simulink model "simulation_ACC_test"  (R2018b)
settings: Solver=ode2  StartTime=0.0  StopTime=90  FixedStep=0.4  RelTol=1e-3
undefined symbols (not defined in the file or in its folder): Delta_T, DiscIntNeverNeededParam, lead_bot_vel_vari, lead_bot_vel_vari_const, sigbuilder_block, timebpt
libraries: commchan3 x11, visionstatistics x4, simulink x3
(part 1 of 3)
settings Model: Creator=UWEcocar  LastModifiedBy=UWEcocar

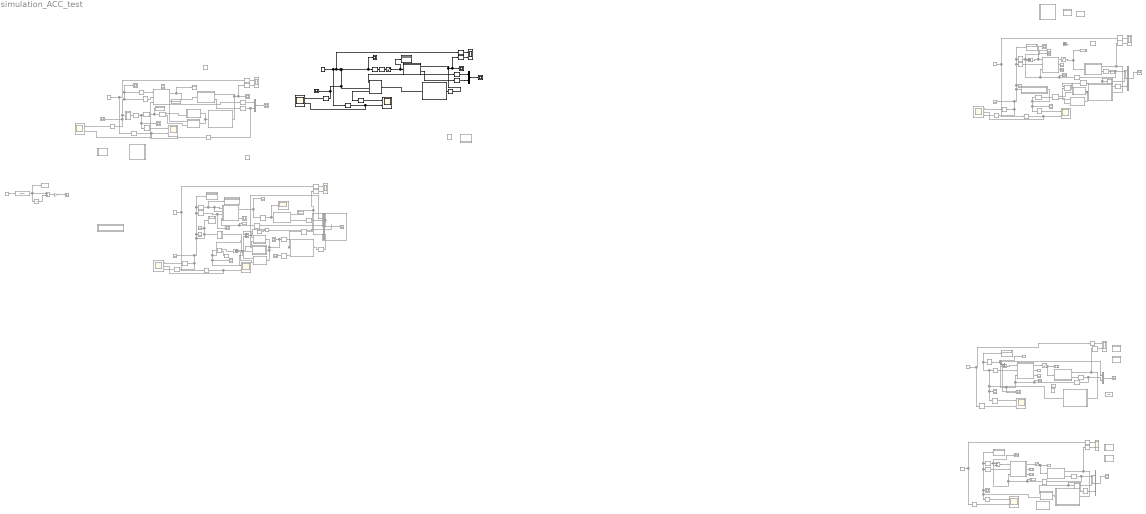
== system simulation_ACC_test ==
  1-D Kalman Filter : Subsystem  Commented=on
  1-D Kalman Filter1 : Subsystem  Commented=on
  1-D Kalman Filter2 : Subsystem  Commented=on
  1-D Kalman Filter3 : Subsystem  Commented=on
  2-D Mean1 : visionstatistics/2-D Mean  Commented=on  run=off  reset_popup=None  directionMode=Each row  dimension=1  treatSBRowAsCol=on  roiEnable=off  roiType=Rectangles  roiPortion=Entire ROI  roiOutput=Individual statistics for each ROI  roiFlag=off  outputDataTypeStr=Inherit: Same as accumulator  outputLastDataTypeStr=Inherit: Same as accumulator  outputMin=[]  outputMax=[]  accumMode=Binary point scaling  accumWordLength=32  accumFracLength=0  accumDataTypeStr=fixdt([],32,0)  accumLastDataTypeStr=fixdt([],32,0)  roundingMode=Floor  overflowMode=off
      settings: SourceProductName=Computer Vision System Toolbox  SourceProductBaseCode=VP
  2-D Mean2 : visionstatistics/2-D Mean  Commented=on  run=off  reset_popup=None  directionMode=Each row  dimension=1  treatSBRowAsCol=on  roiEnable=off  roiType=Rectangles  roiPortion=Entire ROI  roiOutput=Individual statistics for each ROI  roiFlag=off  outputDataTypeStr=Inherit: Same as accumulator  outputLastDataTypeStr=Inherit: Same as accumulator  outputMin=[]  outputMax=[]  accumMode=Binary point scaling  accumWordLength=32  accumFracLength=0  accumDataTypeStr=fixdt([],32,0)  accumLastDataTypeStr=fixdt([],32,0)  roundingMode=Floor  overflowMode=off
      settings: SourceProductName=Computer Vision System Toolbox  SourceProductBaseCode=VP
  2-D Mean3 : visionstatistics/2-D Mean  Commented=on  run=off  reset_popup=None  directionMode=Each row  dimension=1  treatSBRowAsCol=on  roiEnable=off  roiType=Rectangles  roiPortion=Entire ROI  roiOutput=Individual statistics for each ROI  roiFlag=off  outputDataTypeStr=Inherit: Same as accumulator  outputLastDataTypeStr=Inherit: Same as accumulator  outputMin=[]  outputMax=[]  accumMode=Binary point scaling  accumWordLength=32  accumFracLength=0  accumDataTypeStr=fixdt([],32,0)  accumLastDataTypeStr=fixdt([],32,0)  roundingMode=Floor  overflowMode=off
      settings: SourceProductName=Computer Vision System Toolbox  SourceProductBaseCode=VP
  Add : Sum  Commented=on
  Add1 : Sum  Commented=on
  Add2 : Sum  Commented=on  Inputs=+-
  Bus Creator : BusCreator  Inputs=2
  Bus Creator1 : BusCreator  Commented=on  Inputs=2
  Bus Creator2 : BusCreator  Commented=on  Inputs=3
  Bus Creator3 : BusCreator  Commented=on  Inputs=3
  Bus Creator4 : BusCreator  Commented=on  Inputs=3
  Bus Creator5 : BusCreator  Commented=on  Inputs=2
  Camera Sensor1 : Subsystem  Commented=on
  Camera Sensor2 : Subsystem  Commented=on
  Camera Sensor3 : Subsystem  Commented=on
  Camera Sensor4 : Subsystem  Commented=on
  Constant : Constant  Value=[0.4;0]  VectorParams1D=off
  Constant{1..4,7} (5 alike) : Constant  Commented=on  Value=[0.4;0]  VectorParams1D=off
  Constant5 : Constant  Commented=on  Value=0.5
  Constant6 : Constant  Commented=on  Value=0.5
  Delay : Delay  DelayLength=1
  Delay1 : Delay  Commented=on
  Delay2 : Delay  Commented=on
  Delay3 : Delay  Commented=on  DelayLength=1
  Discrete Transfer Fcn : DiscreteTransferFcn  Commented=on  Denominator=[1 0.4]
  Discrete Transfer Fcn1 : DiscreteTransferFcn  Commented=on  Denominator=[1 0.4]
  Discrete Derivative : simulink/Discrete/Discrete Derivative  Commented=on  gainval=1.0  ICPrevScaledInput=0.0  OutMin=[]  OutMax=[]  OutDataType=fixdt(1, 16)  OutScaling=2^-10  DoSatur=off
  Discrete PID Controller : simulink/Continuous/PID Controller  Controller=PI  Form=Parallel  TimeDomain=Discrete-time  SampleTime=-1  IntegratorMethod=Forward Euler  FilterMethod=Forward Euler  ControllerParametersSource=internal  P=0.5  I=0.01  D=0  UseFilter=on  N=100  TunerSelectOption=Transfer Function Based (PID Tuner App)  InitialConditionSource=internal  InitialConditionForIntegrator=0  InitialConditionForFilter=0  DifferentiatorICPrevScaledInput=0  ExternalReset=none  TrackingMode=off  Kt=1  LimitOutput=on  UpperSaturationLimit=0.2  LowerSaturationLimit=-0.2  LinearizeAsGain=off  AntiWindupMode=clamping  Kb=1  POutMin=[]  POutMax=[]  IOutMin=[]  IOutMax=[]  DOutMin=[]  DOutMax=[]  NOutMin=[]  NOutMax=[]  SumOutMin=[]  SumOutMax=[]  SaturationOutMin=[]  SaturationOutMax=[]  PParamMin=[]  PParamMax=[]  IParamMin=[]  IParamMax=[]  DParamMin=[]  DParamMax=[]  NParamMin=[]  NParamMax=[]  KbParamMin=[]  KbParamMax=[]  KtParamMin=[]  KtParamMax=[]  KbOutMin=[]  KbOutMax=[]  KtOutMin=[]  KtOutMax=[]  IntegratorOutMin=[]  IntegratorOutMax=[]  FilterOutMin=[]  FilterOutMax=[]  SumI1OutMin=[]  SumI1OutMax=[]  SumI2OutMin=[]  SumI2OutMax=[]  SumI3OutMin=[]  SumI3OutMax=[]  SumI4OutMin=[]  SumI4OutMax=[]  SumDOutMin=[]  SumDOutMax=[]  DifferentiatorOutMin=[]  DifferentiatorOutMax=[]  FilterDiffOutCoefMin=[]  FilterDiffOutCoefMax=[]  ReciprocalOutMin=[]  ReciprocalOutMax=[]  SumDenOutMin=[]  SumDenOutMax=[]  SumNumOutMin=[]  SumNumOutMax=[]  DivideOutMin=[]  DivideOutMax=[]  IntegratorContinuousStateAttributes=''  IntegratorStateMustResolveToSignalObject=off  IntegratorRTWStateStorageClass=Auto  FilterContinuousStateAttributes=''  FilterStateMustResolveToSignalObject=off  FilterRTWStateStorageClass=Auto  ParallelPVariant=InternalParameters  IdealPVariant=Disabled  IVariant=InternalParameters  DVariant=Disabled  IntegratorVariant=Discrete  SatVariant=Enabled  AWVariant=DiscClampingParallel  PCopyVariant=Disabled  TRVariant=Disabled  FdbkBlocksVariant=Forward  IdealPFdbkVariant=Disabled  SatFdbkVariant=Disabled  DerivativeFilterVariant=Disabled  NVariant=Disabled  NCopyVariant=Disabled_SignalSpec  FilterICVariant=Disabled  IntegratorICVariant=InternalICs  ExternalResetVariant=Disabled  TRSumVariant=Passthrough  SumFdbkVariant=Disabled  SumVariant=Sum_PI
  Discrete PID motor Controller2 : simulink/Continuous/PID Controller  Commented=on  Controller=PI  Form=Parallel  TimeDomain=Discrete-time  SampleTime=-1  IntegratorMethod=Forward Euler  FilterMethod=Forward Euler  ControllerParametersSource=internal  P=0.7813  I=0.0153  D=0  UseFilter=on  N=100  TunerSelectOption=Transfer Function Based (PID Tuner App)  InitialConditionSource=internal  InitialConditionForIntegrator=0  InitialConditionForFilter=0  DifferentiatorICPrevScaledInput=0  ExternalReset=none  TrackingMode=off  Kt=1  LimitOutput=on  UpperSaturationLimit=0.2  LowerSaturationLimit=-0.2  LinearizeAsGain=off  AntiWindupMode=clamping  Kb=1  POutMin=[]  POutMax=[]  IOutMin=[]  IOutMax=[]  DOutMin=[]  DOutMax=[]  NOutMin=[]  NOutMax=[]  SumOutMin=[]  SumOutMax=[]  SaturationOutMin=[]  SaturationOutMax=[]  PParamMin=[]  PParamMax=[]  IParamMin=[]  IParamMax=[]  DParamMin=[]  DParamMax=[]  NParamMin=[]  NParamMax=[]  KbParamMin=[]  KbParamMax=[]  KtParamMin=[]  KtParamMax=[]  KbOutMin=[]  KbOutMax=[]  KtOutMin=[]  KtOutMax=[]  IntegratorOutMin=[]  IntegratorOutMax=[]  FilterOutMin=[]  FilterOutMax=[]  SumI1OutMin=[]  SumI1OutMax=[]  SumI2OutMin=[]  SumI2OutMax=[]  SumI3OutMin=[]  SumI3OutMax=[]  SumI4OutMin=[]  SumI4OutMax=[]  SumDOutMin=[]  SumDOutMax=[]  DifferentiatorOutMin=[]  DifferentiatorOutMax=[]  FilterDiffOutCoefMin=[]  FilterDiffOutCoefMax=[]  ReciprocalOutMin=[]  ReciprocalOutMax=[]  SumDenOutMin=[]  SumDenOutMax=[]  SumNumOutMin=[]  SumNumOutMax=[]  DivideOutMin=[]  DivideOutMax=[]  IntegratorContinuousStateAttributes=''  IntegratorStateMustResolveToSignalObject=off  IntegratorRTWStateStorageClass=Auto  FilterContinuousStateAttributes=''  FilterStateMustResolveToSignalObject=off  FilterRTWStateStorageClass=Auto  ParallelPVariant=InternalParameters  IdealPVariant=Disabled  IVariant=InternalParameters  DVariant=Disabled  IntegratorVariant=Discrete  SatVariant=Enabled  AWVariant=DiscClampingParallel  PCopyVariant=Disabled  TRVariant=Disabled  FdbkBlocksVariant=Forward  IdealPFdbkVariant=Disabled  SatFdbkVariant=Disabled  DerivativeFilterVariant=Disabled  NVariant=Disabled  NCopyVariant=Disabled_SignalSpec  FilterICVariant=Disabled  IntegratorICVariant=InternalICs  ExternalResetVariant=Disabled  TRSumVariant=Passthrough  SumFdbkVariant=Disabled  SumVariant=Sum_PI
  Display{,1..12,14..26} (26 alike) : Display  Commented=on
  Display13 : Display
  Ego vehicle Kinamatics : Subsystem
  Ego vehicle Kinamatics1 : Subsystem  Commented=on
  Ego vehicle Kinamatics2 : Subsystem  Commented=on
  Ego vehicle Kinamatics3 : Subsystem  Commented=on
  Ego vehicle Kinamatics4 : Subsystem  Commented=on
  Ego vehicle Kinamatics5 : Subsystem  Commented=on
  Gain : Gain  Commented=on  Gain=1/Delta_T
  LDS sensor1 : Subsystem  Commented=on
  LDS sensor2 : Subsystem  Commented=on
  LDS sensor3 : Subsystem  Commented=on
  LDS sensor4 : Subsystem  Commented=on
  Lead vehicle trajectory : Subsystem
  Lead vehicle trajectory1 : Subsystem  Commented=on
  Lead vehicle trajectory2 : Subsystem  Commented=on
  Lead vehicle trajectory3 : Subsystem  Commented=on
  Lead vehicle trajectory4 : Subsystem  Commented=on
  Lead vehicle trajectory5 : Subsystem  Commented=on
  MATLAB Function1 : MATLAB Function  Commented=on  TreatAsAtomicUnit=on
  MATLAB Function10 : MATLAB Function  Commented=on  TreatAsAtomicUnit=on
  MATLAB Function11 : MATLAB Function  Commented=on  TreatAsAtomicUnit=on
  MATLAB Function12 : MATLAB Function  Commented=on  TreatAsAtomicUnit=on
  MATLAB Function13 : MATLAB Function  Commented=on  TreatAsAtomicUnit=on
  MATLAB Function2 : MATLAB Function  Commented=on  TreatAsAtomicUnit=on
  MATLAB Function3 : MATLAB Function  Commented=on  TreatAsAtomicUnit=on
  MATLAB Function4 : MATLAB Function  Commented=on  TreatAsAtomicUnit=on
  MATLAB Function5 : MATLAB Function  Commented=on  TreatAsAtomicUnit=on
  MATLAB Function6 : MATLAB Function  Commented=on  TreatAsAtomicUnit=on
  MATLAB Function7 : MATLAB Function  Commented=on  TreatAsAtomicUnit=on
  MATLAB Function8 : MATLAB Function  Commented=on  TreatAsAtomicUnit=on
  MATLAB Function9 : MATLAB Function  Commented=on  TreatAsAtomicUnit=on
  Matrix Concatenate1 : Concatenate  Commented=on  Mode=Multidimensional array  ConcatenateDimension=2
  Matrix Concatenate2 : Concatenate  Commented=on  Mode=Multidimensional array  ConcatenateDimension=2
  Matrix Concatenate3 : Concatenate  Commented=on  Mode=Multidimensional array  ConcatenateDimension=2
  Memory : Memory  Commented=on
  Multiply : Product  Commented=on
  Multiply1 : Product  Commented=on
  New_1d_kalman_filter : Subsystem  Commented=on
  New_1d_kalman_filter2 : Subsystem  Commented=on
  Saturation : Saturate  Commented=on  UpperLimit=0.2  LowerLimit=-0.2
  Saturation1 : Saturate  Commented=on  UpperLimit=0.2  LowerLimit=-0.2
  Saturation2 : Saturate  UpperLimit=0.2  LowerLimit=0
  Saturation3 : Saturate  Commented=on  UpperLimit=0.2  LowerLimit=0
  Scope{,2..3,5} (4 alike) : Scope
  Scope1 : Scope  NumInputPorts=2
  Scope{7,10,12,16..17,19,25..26,32,40,43,46} (12 alike) : Scope  Commented=on  NumInputPorts=2
  Scope{6,9,11,13..15,18,20..22,24,27..29,31,33..39,41..42,44..45,47} (27 alike) : Scope  Commented=on
  Scope23 : Scope  Commented=on  NumInputPorts=3
  Scope30 : Scope  Commented=on  NumInputPorts=3
  Scope4 : Scope  NumInputPorts=2
  Scope8 : Scope  NumInputPorts=2
  Selector{1..4,6..7,12} (7 alike) : Selector  InputPortWidth=2  IndexOptions=Index vector (dialog)  Indices=[1]  OutputSizes=1
  Selector{8..11,13..14,16..19,21..22,25,27..28,30..34,36,38..40,42..47,49..51,53..54,56} (36 alike) : Selector  Commented=on  InputPortWidth=2  IndexOptions=Index vector (dialog)  Indices=[1]  OutputSizes=1
  Selector{15,20,23..24,26,29,35,37,41,48,52,55} (12 alike) : Selector  Commented=on  InputPortWidth=2  IndexOptions=Index vector (dialog)  Indices=[2]  OutputSizes=1
  Selector5 : Selector  InputPortWidth=2  IndexOptions=Index vector (dialog)  Indices=[2]  OutputSizes=1
  Sensor Fusion : Subsystem
  Subtract{,1..3} (4 alike) : Sum  Commented=on  Inputs=+-
  Sum : Sum  Inputs=|-+
  Transfer Fcn : TransferFcn  Commented=on  Denominator=[4 1]
  Transfer Fcn1 : TransferFcn  Commented=on  Denominator=[0.2 1]
  Transport Delay{,1..2,4..5} (5 alike) : TransportDelay  Commented=on  DelayTime=0.8
  Transport Delay3 : TransportDelay  Commented=on  DelayTime=0.4
  Transport Delay9 : TransportDelay  Commented=on  DelayTime=0.4
  Unit Delay : UnitDelay  Commented=on  SampleTime=-1
  Unit Delay1 : UnitDelay  Commented=on  SampleTime=-1
  V_lead2 : Constant  Commented=on
  combined sensor4 : Subsystem  Commented=on
  wires:
  Sum/1 -> Scope2/1, Selector1/1
  Constant/1 -> Selector6/1, Selector2/1, Sum/1
  Selector1/1 -> Discrete PID Controller/1
  Selector3/1 -> Scope1/2
  Selector2/1 -> Scope1/1
  Selector5/1 -> Bus Creator/1  "lead vehicle speed"
  Selector4/1 -> Bus Creator/2  "ego vehicle speed"
  Bus Creator/1 -> Scope5/1
  Selector6/1 -> Scope4/2, Scope8/2  "safe distance = 0.4m"
  Selector7/1 -> Scope8/1  "relative distance measured by sensor"
  Selector14/1 -> Scope17/1  "relative distance measured by sensor"
  MATLAB Function4/1(accel_new) -> Saturation/1  "ego vehicle speed"
  Constant2/1 -> Selector13/1, Selector9/1
  Selector10/1 -> Scope10/2
  Selector13/1 -> Scope17/2  "safe distance = 0.4m"
  Bus Creator1/1 -> Scope14/1
  Selector9/1 -> Scope10/1
  Lead vehicle trajectory2/1(Lead vehicle traject. and ego vehicle state out) -> Display/1, Selector15/1, Selector8/1, Selector14/1, Scope15/1
  Selector8/1 -> MATLAB Function4/2(rel_posx)  "relative distance"
  Selector15/1 -> Scope16/1, Subtract/1, Display3/1, Bus Creator1/1  "lead velocity"
  MATLAB Function4/2(stat) -> Display1/1
  Ego vehicle Kinamatics/1(Output for sensor feedback) -> Delay/1, Selector3/1, Scope/1
  Ego vehicle Kinamatics/2(ego vehicle speed) -> Selector4/1
  Selector12/1 -> Scope4/1  "relative distance estimated by kalman filter through sensor"
  MATLAB Function4/3(x) -> Display2/1
  Ego vehicle Kinamatics2/2(ego vehicle speed) -> Selector11/1
  Ego vehicle Kinamatics2/1(Output for sensor feedback) -> Selector10/1, Lead vehicle trajectory2/1(ego vehicle input)
  Subtract/1 -> MATLAB Function4/1(rel_velx)  "relative velocity"
  Selector11/1 -> Transport Delay/1, Bus Creator1/2  "ego vehicle speed"
  Saturation/1 -> Display4/1, Ego vehicle Kinamatics2/1(Controller input (x; vx))
  Saturation1/1 -> Display10/1, Ego vehicle Kinamatics1/1(Controller input (x; vx))
  Selector17/1 -> Transport Delay1/1, Bus Creator2/2  "ego vehicle speed"
  Ego vehicle Kinamatics1/1(Output for sensor feedback) -> Selector16/1, Lead vehicle trajectory1/1(ego vehicle input)
  Selector21/1 -> MATLAB Function6/2(rel_posx)  "relative distance"
  MATLAB Function6/3(x) -> Display8/1
  Subtract1/1 -> MATLAB Function6/1(rel_velx)  "relative velocity"
  Bus Creator2/1 -> Scope9/1
  Ego vehicle Kinamatics1/2(ego vehicle speed) -> Selector17/1
  Selector22/1 -> Scope7/1
  Selector16/1 -> Scope7/2
  MATLAB Function6/1(accel_new) -> Saturation1/1  "ego vehicle speed"
  Selector18/1 -> Scope12/2  "safe distance = 0.4m"
  Selector20/1 -> Display9/1, Subtract1/1  "lead velocity"
  Selector19/1 -> Scope12/1  "relative distance measured by sensor with noise"
  MATLAB Function6/2(stat) -> Display7/1
  Constant1/1 -> Selector18/1, Selector22/1
  Camera Sensor1/2(Sensor Output) -> Selector19/1, Scope11/1, Display6/1, Selector20/1, Selector21/1
  Lead vehicle trajectory1/1(Lead vehicle traject. and ego vehicle state out) -> Camera Sensor1/1(Traject. input)
  Camera Sensor1/1(Act lead vehicle speed) -> Selector26/1, Selector25/1
  Transport Delay/1 -> MATLAB Function4/3(vel_egox), Scope16/2, Subtract/2, Display5/1
  Transport Delay1/1 -> Display11/1, MATLAB Function6/3(vel_egox), Subtract1/2
  Delay/1 -> Lead vehicle trajectory/1(ego vehicle input)
  Selector25/1 -> Bus Creator2/1  "estimated distance by sensor"
  Selector26/1 -> Bus Creator2/3  "lead vehicle speed"
  Selector38/1 -> MATLAB Function12/2(rel_posx)  "relative distance"
  Subtract3/1 -> Scope13/1, Display12/1, MATLAB Function12/1(rel_velx)  "relative velocity"
  MATLAB Function12/2(stat) -> Display21/1
  MATLAB Function12/1(accel_new) -> Saturation3/1  "ego vehicle speed"
  Selector41/1 -> Bus Creator4/3  "lead vehicle speed"
  Ego vehicle Kinamatics3/2(ego vehicle speed) -> Selector34/1
  Selector33/1 -> Scope26/2
  Selector37/1 -> Display23/1, Subtract3/1  "lead velocity"
  MATLAB Function12/3(x) -> Display22/1
  Selector34/1 -> Discrete Transfer Fcn/1
  Selector39/1 -> Scope26/1
  Bus Creator4/1 -> Scope27/1
  Transport Delay4/1 -> Display19/1, MATLAB Function12/3(vel_egox), Subtract3/2
  Lead vehicle trajectory4/1(Lead vehicle traject. and ego vehicle state out) -> LDS sensor3/1(Traject. input), Camera Sensor3/1(Traject. input)
  Selector40/1 -> Bus Creator4/1  "estimated distance by sensor"
  Ego vehicle Kinamatics3/1(Output for sensor feedback) -> Selector33/1, Lead vehicle trajectory4/1(ego vehicle input)
  Camera Sensor3/1(Act lead vehicle speed) -> Matrix Concatenate3/1
  Selector43/1 -> Scope30/2, Scope32/2  "safe distance = 0.4m"
  2-D Mean2/1 -> 1-D Kalman Filter1/1(Sensor Input), Scope31/1, Selector44/1
  Selector44/1 -> Scope32/1  "relative distance measured by sensor"
  Selector42/1 -> Scope30/1  "relative distance estimated kalman filter"
  Matrix Concatenate2/1 -> 2-D Mean2/1
  Constant4/1 -> Selector43/1, Selector39/1
  LDS sensor3/2(Sensor Output) -> Matrix Concatenate2/2
  Camera Sensor3/2(Sensor Output) -> Matrix Concatenate2/1
  LDS sensor3/1(Act lead vehicle speed) -> Matrix Concatenate3/2
  Matrix Concatenate3/1 -> 2-D Mean3/1
  2-D Mean3/1 -> Selector41/1, Selector40/1
  1-D Kalman Filter1/1(measurement and estimated velocity) -> Selector23/1, Selector42/1, Scope29/1, Scope28/1, Selector38/1, Selector37/1, Display20/1
  Discrete PID Controller/1 -> Saturation2/1
  Saturation3/1 -> Ego vehicle Kinamatics3/1(Controller input (x; vx)), Display18/1  "opt_cmd"
  Selector23/1 -> Scope30/3  "relative velocity estimated kalman filter"
  Subtract2/1 -> ?
  Discrete Transfer Fcn/1 -> Transport Delay4/1, Bus Creator4/2  "ego vehicle speed"
  Selector24/1 -> Scope23/3  "relative velocity estimated kalman filter"
  MATLAB Function9/1(accel_new) -> Transport Delay9/1, Scope18/1  "opt_cmd"
  Ego vehicle Kinamatics4/1(Output for sensor feedback) -> Transport Delay5/1, Selector27/1
  Selector45/1 -> Scope23/2, Scope25/2  "safe distance = 0.4m"
  Lead vehicle trajectory3/1(Lead vehicle traject. and ego vehicle state out) -> Selector35/1, Selector47/1, Selector48/1
  Camera Sensor2/2(Sensor Output) -> Add1/1
  Selector31/1 -> Scope19/1
  Transport Delay3/1 -> MATLAB Function9/4(vel_egox), Display16/1
  Constant3/1 -> Selector45/1, Selector31/1
  Selector30/1 -> Scope38/1, MATLAB Function9/3(rel_posx)  "relative distance"
  Camera Sensor2/1(sensor rel. distance) -> Add/1
  Selector36/1 -> Scope23/1  "relative distance estimated kalman filter"
  Bus Creator3/1 -> Scope20/1
  LDS sensor2/2(Sensor Output) -> Add1/2
  LDS sensor2/1(sensor rel. distance) -> Add/2
  Add/1 -> Multiply/1
  Multiply/1 -> ?  "estimated distance by sensor"
  Selector29/1 -> MATLAB Function9/2(rel_velx), MATLAB Function9/1(lead_velocity), Display26/1  "lead velocity"
  Selector27/1 -> Scope19/2
  Add1/1 -> Multiply1/1
  Selector35/1 -> Bus Creator3/3  "lead vehicle speed"
  Multiply1/1 -> Scope24/1  "relative distance measured by sensor"
  Selector28/1 -> Transport Delay3/1, Bus Creator3/2  "ego vehicle speed"
  Selector47/1 -> combined sensor4/1(Traject. input), LDS sensor2/1(Traject. input), Camera Sensor2/1(Traject. input), Scope33/1  "relative distance"
  Selector48/1 -> Scope34/1
  Constant5/1 -> Multiply/2
  Constant6/1 -> Multiply1/2
  MATLAB Function9/2(stat) -> Scope37/1
  Ego vehicle Kinamatics4/2(ego vehicle speed) -> Selector28/1  "ego vehicle speed"
  Transport Delay9/1 -> Scope36/1, Ego vehicle Kinamatics4/1(Controller input (x; vx))
  combined sensor4/1(sensor rel. distance) -> Bus Creator3/1  "estimated distance by sensor"
  combined sensor4/2(Sensor Output) -> New_1d_kalman_filter2/1(In1), Scope25/1  "relative distance measured by sensor"
  New_1d_kalman_filter2/1(Out1) -> Selector24/1, Selector36/1, Scope22/1, Scope21/1, Selector30/1, Selector29/1, Display17/1, Display14/1, Scope35/1  "matlab kalman"
  Transport Delay5/1 -> Lead vehicle trajectory3/1(ego vehicle input)
  LDS sensor4/2(Sensor Output) -> Matrix Concatenate1/1
  Selector46/1 -> Scope43/1  "relative distance estimated be kalman filter through sensor"
  Selector51/1 -> Delay3/1, Bus Creator5/2  "ego vehicle speed"
  Selector49/1 -> Scope40/1
  Selector53/1 -> Scope43/2, Scope46/2  "safe distance = 0.4m"
  Ego vehicle Kinamatics5/1(Output for sensor feedback) -> Lead vehicle trajectory5/1(ego vehicle input), Selector50/1, Scope39/1
  Selector52/1 -> Bus Creator5/1  "lead vehicle speed"
  Camera Sensor4/2(Sensor Output) -> Matrix Concatenate1/2
  Selector32/1 -> MATLAB Function13/2(rel_posx)
  Ego vehicle Kinamatics5/2(ego vehicle speed) -> Selector51/1
  Selector54/1 -> Scope46/1  "relative distance measured by sensor"
  Matrix Concatenate1/1 -> Display25/1, 2-D Mean1/1
  Bus Creator5/1 -> Scope44/1
  Selector50/1 -> Scope40/2
  Constant7/1 -> Selector53/1, Selector49/1
  Camera Sensor4/1(Act lead vehicle speed) -> Selector52/1
  Lead vehicle trajectory5/1(Lead vehicle traject. and ego vehicle state out) -> LDS sensor4/1(Traject. input), Camera Sensor4/1(Traject. input)
  Selector55/1 -> MATLAB Function13/1(rel_velx)  "relative velocity estimated by kalman"
  MATLAB Function13/2(stat) -> Display24/1
  New_1d_kalman_filter/1(Out1) -> Selector32/1, Selector55/1, Scope41/1, Selector46/1, Scope42/1
  2-D Mean1/1 -> Selector56/1, Selector54/1, Scope45/1
  Selector56/1 -> New_1d_kalman_filter/1(In1)
  Saturation2/1 -> Display13/1, Ego vehicle Kinamatics/1(Controller input (x; vx))
  Sensor Fusion/3(kalman out) -> Sum/2, Scope3/1, Selector12/1
  Lead vehicle trajectory/1(Lead vehicle traject. and ego vehicle state out) -> Sensor Fusion/1(simulated input)
  Sensor Fusion/1(lead vehicle speed) -> Selector5/1
  Sensor Fusion/4(sensor out) -> Selector7/1
  MATLAB Function13/1(accel_new) -> Ego vehicle Kinamatics5/1(Controller input (vx)), Display15/1
  Delay3/1 -> MATLAB Function13/3(vel_egox)
  Transfer Fcn1/1 -> Discrete Derivative/1, Add2/1, Unit Delay1/1  "V_following"
  V_lead2/1 -> Transfer Fcn1/1
  Gain/1 -> Scope6/1
  Unit Delay1/1 -> Add2/2
  Add2/1 -> Gain/1

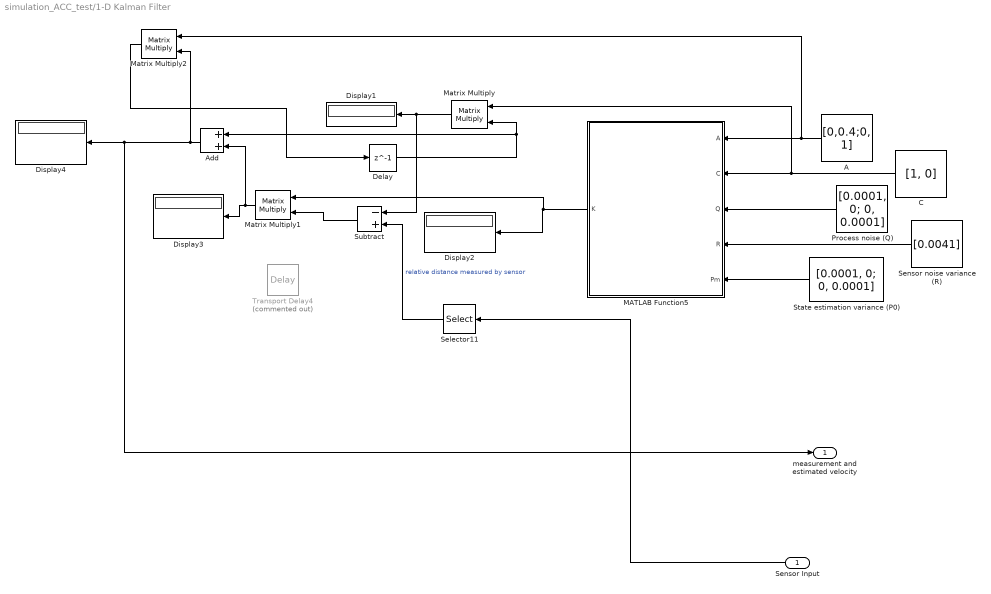
== system simulation_ACC_test/1-D Kalman Filter ==
  Sensor Input : Inport
  A : Constant  Value=[0,0.4;0, 1]  VectorParams1D=off
  Add : Sum
  C : Constant  Value=[1, 0]  VectorParams1D=off
  Delay : Delay  DelayLength=1
  Display{1..4} (4 alike) : Display
  MATLAB Function5 : MATLAB Function  TreatAsAtomicUnit=on
  Matrix Multiply : Product  Multiplication=Matrix(*)
  Matrix Multiply1 : Product  Multiplication=Matrix(*)
  Matrix Multiply2 : Product  Multiplication=Matrix(*)
  Process noise (Q) : Constant  Value=|  VectorParams1D=off
      | [0.0001, 0;
      | 0, 0.0001]
  Selector11 : Selector  InputPortWidth=2  IndexOptions=Index vector (dialog)  Indices=[1]  OutputSizes=1
  Sensor noise variance (R) : Constant  Value=[0.0041]  VectorParams1D=off
  State estimation variance (P0) : Constant  Value=[0.0001, 0; 0, 0.0001]  VectorParams1D=off
  Subtract : Sum  Inputs=-+
  Transport Delay4 : TransportDelay  Commented=on  DelayTime=0.4
  measurement and estimated velocity : Outport
  wires:
  MATLAB Function5/1(K) -> Matrix Multiply1/1, Display2/1
  Matrix Multiply1/1 -> Add/2, Display3/1
  Selector11/1 -> Subtract/2  "relative distance measured by sensor"
  Matrix Multiply2/1 -> Delay/1
  A/1 -> Matrix Multiply2/1, MATLAB Function5/1(A)
  State estimation variance (P0)/1 -> MATLAB Function5/5(Pm)
  Add/1 -> Matrix Multiply2/2, measurement and estimated velocity/1, Display4/1
  C/1 -> Matrix Multiply/1, MATLAB Function5/2(C)
  Process noise (Q)/1 -> MATLAB Function5/3(Q)
  Matrix Multiply/1 -> Subtract/1, Display1/1
  Sensor noise variance (R)/1 -> MATLAB Function5/4(R)
  Sensor Input/1 -> Selector11/1
  Subtract/1 -> Matrix Multiply1/2
  Delay/1 -> Add/1, Matrix Multiply/2

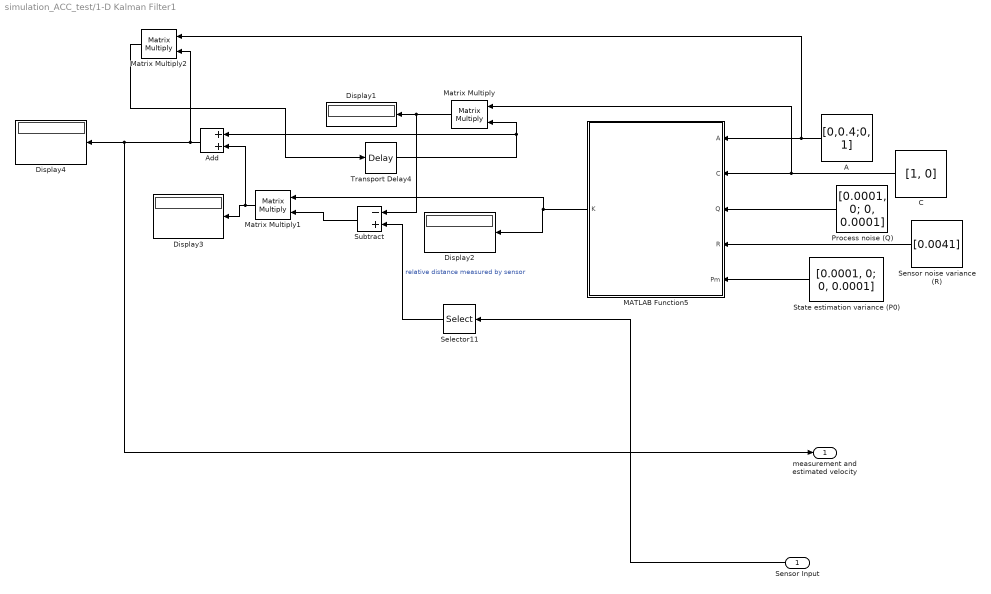
== system simulation_ACC_test/1-D Kalman Filter1 ==
  Sensor Input : Inport
  A : Constant  Value=[0,0.4;0, 1]  VectorParams1D=off
  Add : Sum
  C : Constant  Value=[1, 0]  VectorParams1D=off
  Display{1..4} (4 alike) : Display
  MATLAB Function5 : MATLAB Function  TreatAsAtomicUnit=on
  Matrix Multiply : Product  Multiplication=Matrix(*)
  Matrix Multiply1 : Product  Multiplication=Matrix(*)
  Matrix Multiply2 : Product  Multiplication=Matrix(*)
  Process noise (Q) : Constant  Value=|  VectorParams1D=off
      | [0.0001, 0;
      | 0, 0.0001]
  Selector11 : Selector  InputPortWidth=2  IndexOptions=Index vector (dialog)  Indices=[1]  OutputSizes=1
  Sensor noise variance (R) : Constant  Value=[0.0041]  VectorParams1D=off
  State estimation variance (P0) : Constant  Value=[0.0001, 0; 0, 0.0001]  VectorParams1D=off
  Subtract : Sum  Inputs=-+
  Transport Delay4 : TransportDelay  DelayTime=0.4
  measurement and estimated velocity : Outport
  wires:
  MATLAB Function5/1(K) -> Matrix Multiply1/1, Display2/1
  Matrix Multiply1/1 -> Add/2, Display3/1
  Selector11/1 -> Subtract/2  "relative distance measured by sensor"
  Matrix Multiply2/1 -> Transport Delay4/1
  A/1 -> Matrix Multiply2/1, MATLAB Function5/1(A)
  State estimation variance (P0)/1 -> MATLAB Function5/5(Pm)
  Add/1 -> Matrix Multiply2/2, measurement and estimated velocity/1, Display4/1
  C/1 -> Matrix Multiply/1, MATLAB Function5/2(C)
  Process noise (Q)/1 -> MATLAB Function5/3(Q)
  Matrix Multiply/1 -> Subtract/1, Display1/1
  Sensor noise variance (R)/1 -> MATLAB Function5/4(R)
  Sensor Input/1 -> Selector11/1
  Subtract/1 -> Matrix Multiply1/2
  Transport Delay4/1 -> Add/1, Matrix Multiply/2

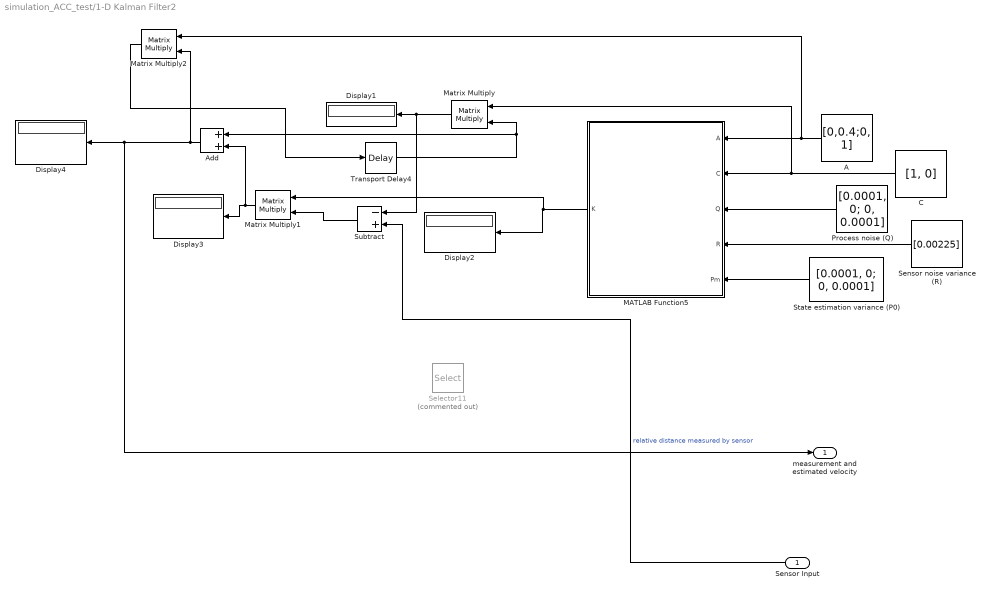
== system simulation_ACC_test/1-D Kalman Filter2 ==
  Sensor Input : Inport
  A : Constant  Value=[0,0.4;0, 1]  VectorParams1D=off
  Add : Sum
  C : Constant  Value=[1, 0]  VectorParams1D=off
  Display{1..4} (4 alike) : Display
  MATLAB Function5 : MATLAB Function  TreatAsAtomicUnit=on
  Matrix Multiply : Product  Multiplication=Matrix(*)
  Matrix Multiply1 : Product  Multiplication=Matrix(*)
  Matrix Multiply2 : Product  Multiplication=Matrix(*)
  Process noise (Q) : Constant  Value=|  VectorParams1D=off
      | [0.0001, 0;
      | 0, 0.0001]
  Selector11 : Selector  Commented=on  InputPortWidth=2  IndexOptions=Index vector (dialog)  Indices=[1]  OutputSizes=1
  Sensor noise variance (R) : Constant  Value=[0.00225]  VectorParams1D=off
  State estimation variance (P0) : Constant  Value=[0.0001, 0; 0, 0.0001]  VectorParams1D=off
  Subtract : Sum  Inputs=-+
  Transport Delay4 : TransportDelay  DelayTime=0.4
  measurement and estimated velocity : Outport
  wires:
  MATLAB Function5/1(K) -> Matrix Multiply1/1, Display2/1
  Matrix Multiply1/1 -> Add/2, Display3/1
  Sensor Input/1 -> Subtract/2  "relative distance measured by sensor"
  Matrix Multiply2/1 -> Transport Delay4/1
  A/1 -> Matrix Multiply2/1, MATLAB Function5/1(A)
  State estimation variance (P0)/1 -> MATLAB Function5/5(Pm)
  Add/1 -> Matrix Multiply2/2, measurement and estimated velocity/1, Display4/1
  C/1 -> Matrix Multiply/1, MATLAB Function5/2(C)
  Process noise (Q)/1 -> MATLAB Function5/3(Q)
  Matrix Multiply/1 -> Subtract/1, Display1/1
  Sensor noise variance (R)/1 -> MATLAB Function5/4(R)
  Subtract/1 -> Matrix Multiply1/2
  Transport Delay4/1 -> Add/1, Matrix Multiply/2

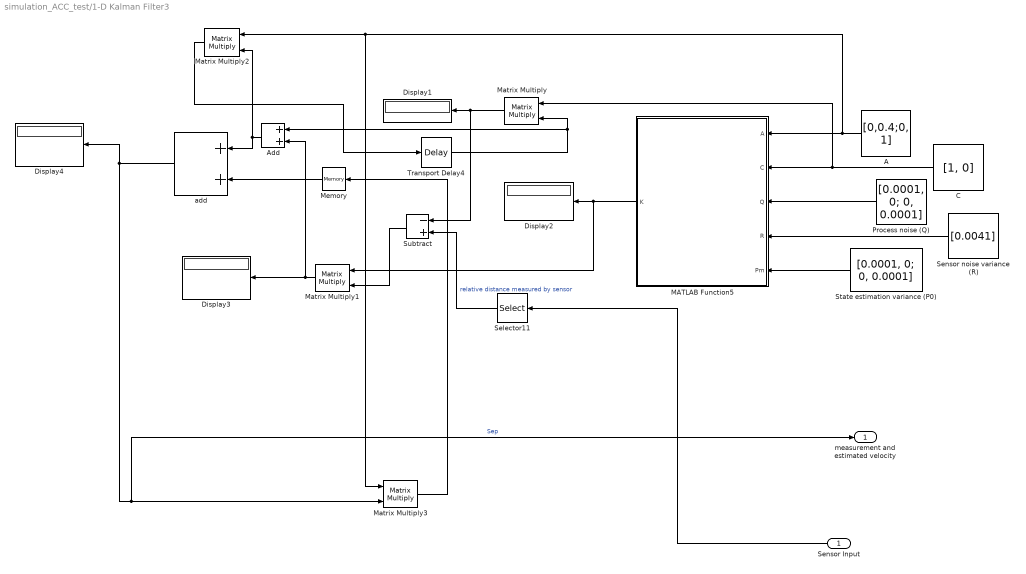
== system simulation_ACC_test/1-D Kalman Filter3 ==
  Sensor Input : Inport
  A : Constant  Value=[0,0.4;0, 1]  VectorParams1D=off
  Add : Sum
  C : Constant  Value=[1, 0]  VectorParams1D=off
  Display{1..4} (4 alike) : Display
  MATLAB Function5 : MATLAB Function  TreatAsAtomicUnit=on
  Matrix Multiply{,1..3} (4 alike) : Product  Multiplication=Matrix(*)
  Memory : Memory  InitialCondition=[0, 0]'
  Process noise (Q) : Constant  Value=|  VectorParams1D=off
      | [0.0001, 0;
      | 0, 0.0001]
  Selector11 : Selector  InputPortWidth=2  IndexOptions=Index vector (dialog)  Indices=[1]  OutputSizes=1
  Sensor noise variance (R) : Constant  Value=[0.0041]  VectorParams1D=off
  State estimation variance (P0) : Constant  Value=[0.0001, 0; 0, 0.0001]  VectorParams1D=off
  Subtract : Sum  Inputs=-+
  Transport Delay4 : TransportDelay  DelayTime=0.4
  add : Sum
  measurement and estimated velocity : Outport
  wires:
  MATLAB Function5/1(K) -> Matrix Multiply1/1, Display2/1
  Matrix Multiply1/1 -> Add/2, Display3/1
  Selector11/1 -> Subtract/2  "relative distance measured by sensor"
  Matrix Multiply2/1 -> Transport Delay4/1
  A/1 -> Matrix Multiply2/1, Matrix Multiply3/1, MATLAB Function5/1(A)
  State estimation variance (P0)/1 -> MATLAB Function5/5(Pm)
  Add/1 -> add/1, Matrix Multiply2/2
  C/1 -> Matrix Multiply/1, MATLAB Function5/2(C)
  Process noise (Q)/1 -> MATLAB Function5/3(Q)
  Matrix Multiply/1 -> Subtract/1, Display1/1
  Sensor noise variance (R)/1 -> MATLAB Function5/4(R)
  Sensor Input/1 -> Selector11/1
  Subtract/1 -> Matrix Multiply1/2
  Transport Delay4/1 -> Add/1, Matrix Multiply/2
  Matrix Multiply3/1 -> Memory/1
  add/1 -> Display4/1, measurement and estimated velocity/1, Matrix Multiply3/2  "Sep"
  Memory/1 -> add/2

== system simulation_ACC_test/Camera Sensor1 ==
  Traject. input : Inport
  AWGN Channel : commchan3/AWGN Channel  InputProcessing=Columns as channels (frame based)  seed=67  noiseMode="Signal to noise ratio  (SNR)"  EbNodB=100  EsNodB=10  SNRdB=19  bitsPerSym=1  Ps=1  Tsym=0.4  variance=1
  C : Constant  Value="[1, 0;    0, 1]"  VectorParams1D=off
  Product2 : Product  Multiplication=Matrix(*)
  Scope4 : Scope
  Scope7 : Scope
  Act lead vehicle speed : Outport
  Sensor Output : Outport  Port=2
  wires:
  Traject. input/1 -> Product2/2, Scope4/1  "Trajectory input"
  AWGN Channel/1 -> Sensor Output/1  "Sensor output"
  C/1 -> Product2/1
  Product2/1 -> Act lead vehicle speed/1, AWGN Channel/1, Scope7/1  "Actual Lead vehicle speed"

== system simulation_ACC_test/Camera Sensor2 ==
  Traject. input : Inport
  AWGN Channel : commchan3/AWGN Channel  InputProcessing=Columns as channels (frame based)  seed=67  noiseMode="Signal to noise ratio  (SNR)"  EbNodB=100  EsNodB=10  SNRdB=19  bitsPerSym=1  Ps=1  Tsym=0.4  variance=1
  C : Constant  Commented=on  Value=[1, 0]  VectorParams1D=off
  Scope4 : Scope
  Scope7 : Scope
  sensor rel. distance : Outport
  Sensor Output : Outport  Port=2
  wires:
  Traject. input/1 -> sensor rel. distance/1, AWGN Channel/1, Scope7/1, Scope4/1  "Trajectory input"
  AWGN Channel/1 -> Sensor Output/1  "Sensor output"

== system simulation_ACC_test/Camera Sensor3 ==
  Traject. input : Inport
  AWGN Channel : commchan3/AWGN Channel  InputProcessing=Columns as channels (frame based)  seed=67  noiseMode="Signal to noise ratio  (SNR)"  EbNodB=100  EsNodB=10  SNRdB=19  bitsPerSym=1  Ps=1  Tsym=0.4  variance=1
  C : Constant  Value="[1, 0;    0, 1]"  VectorParams1D=off
  Product2 : Product  Multiplication=Matrix(*)
  Scope4 : Scope
  Scope7 : Scope
  Act lead vehicle speed : Outport
  Sensor Output : Outport  Port=2
  wires:
  Traject. input/1 -> Product2/2, Scope4/1  "Trajectory input"
  AWGN Channel/1 -> Sensor Output/1  "Sensor output"
  C/1 -> Product2/1
  Product2/1 -> Act lead vehicle speed/1, AWGN Channel/1, Scope7/1  "Actual Lead vehicle speed"

== system simulation_ACC_test/Camera Sensor4 ==
  Traject. input : Inport
  AWGN Channel : commchan3/AWGN Channel  InputProcessing=Columns as channels (frame based)  seed=67  noiseMode="Signal to noise ratio  (SNR)"  EbNodB=100  EsNodB=10  SNRdB=19  bitsPerSym=1  Ps=1  Tsym=0.4  variance=1
  C : Constant  Value="[1, 0;    0, 1]"  VectorParams1D=off
  Product2 : Product  Multiplication=Matrix(*)
  Scope4 : Scope
  Scope7 : Scope
  Act lead vehicle speed : Outport
  Sensor Output : Outport  Port=2
  wires:
  Traject. input/1 -> Product2/2, Scope4/1  "Trajectory input"
  C/1 -> Product2/1
  Product2/1 -> Act lead vehicle speed/1, AWGN Channel/1, Scope7/1  "Actual Lead vehicle speed"
  AWGN Channel/1 -> Sensor Output/1  "Sensor output"

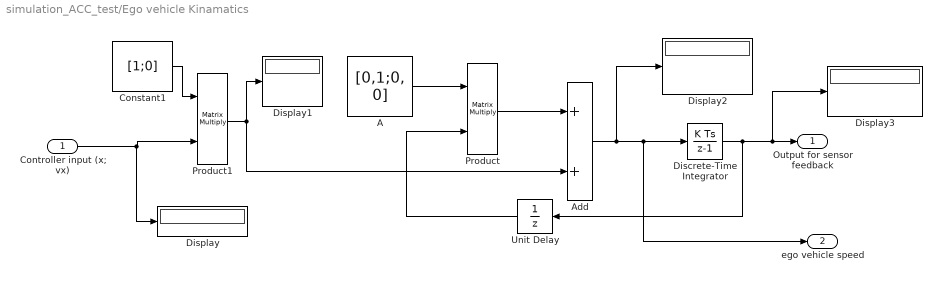
== system simulation_ACC_test/Ego vehicle Kinamatics ==
  Controller input (x; vx) : Inport
  A : Constant  Value=[0,1;0, 0]  VectorParams1D=off
  Add : Sum
  Constant1 : Constant  Value=[1;0]  VectorParams1D=off
  Discrete-Time Integrator : DiscreteIntegrator  InitialCondition=[0;0]  SampleTime=-1  ICPrevOutput=DiscIntNeverNeededParam  ICPrevScaledInput=DiscIntNeverNeededParam
  Display{,1..3} (4 alike) : Display
  Product : Product  Multiplication=Matrix(*)
  Product1 : Product  Multiplication=Matrix(*)
  Unit Delay : UnitDelay  SampleTime=-1
  Output for sensor feedback : Outport
  ego vehicle speed : Outport  Port=2
  wires:
  Discrete-Time Integrator/1 -> Unit Delay/1, Display3/1, Output for sensor feedback/1
  A/1 -> Product/1
  Controller input (x; vx)/1 -> Display/1, Product1/2
  Product1/1 -> Display1/1, Add/2
  Add/1 -> Display2/1, ego vehicle speed/1, Discrete-Time Integrator/1
  Product/1 -> Add/1
  Constant1/1 -> Product1/1
  Unit Delay/1 -> Product/2

== system simulation_ACC_test/Ego vehicle Kinamatics1 ==
  Controller input (x; vx) : Inport
  A : Constant  Value=[0,1;0, 0]  VectorParams1D=off
  Add : Sum
  Constant1 : Constant  Value=[1;0]  VectorParams1D=off
  Discrete-Time Integrator : DiscreteIntegrator  InitialCondition=[0;0]  SampleTime=-1  ICPrevOutput=DiscIntNeverNeededParam  ICPrevScaledInput=DiscIntNeverNeededParam
  Product : Product  Multiplication=Matrix(*)
  Product1 : Product  Multiplication=Matrix(*)
  Scope3 : Scope
  Unit Delay : UnitDelay  SampleTime=-1
  Output for sensor feedback : Outport
  ego vehicle speed : Outport  Port=2
  wires:
  Discrete-Time Integrator/1 -> Unit Delay/1, Output for sensor feedback/1
  A/1 -> Product/1
  Controller input (x; vx)/1 -> Product1/2
  Product1/1 -> Scope3/1, Add/2
  Add/1 -> ego vehicle speed/1, Discrete-Time Integrator/1
  Product/1 -> Add/1
  Constant1/1 -> Product1/1
  Unit Delay/1 -> Product/2

== system simulation_ACC_test/Ego vehicle Kinamatics2 ==
  Controller input (x; vx) : Inport
  A : Constant  Value=[0,1;0, 0]  VectorParams1D=off
  Add : Sum
  Constant1 : Constant  Value=[1;0]  VectorParams1D=off
  Discrete-Time Integrator : DiscreteIntegrator  InitialCondition=[0;0]  SampleTime=-1  ICPrevOutput=DiscIntNeverNeededParam  ICPrevScaledInput=DiscIntNeverNeededParam
  Memory : Memory  Commented=on
  Product : Product  Multiplication=Matrix(*)
  Product1 : Product  Multiplication=Matrix(*)
  Scope3 : Scope
  Unit Delay : UnitDelay  SampleTime=-1
  Output for sensor feedback : Outport
  ego vehicle speed : Outport  Port=2
  wires:
  Discrete-Time Integrator/1 -> Unit Delay/1, Output for sensor feedback/1
  A/1 -> Product/1
  Controller input (x; vx)/1 -> Product1/2
  Product1/1 -> Scope3/1, Add/2
  Product/1 -> Add/1
  Constant1/1 -> Product1/1
  Unit Delay/1 -> Product/2
  Add/1 -> ego vehicle speed/1, Discrete-Time Integrator/1

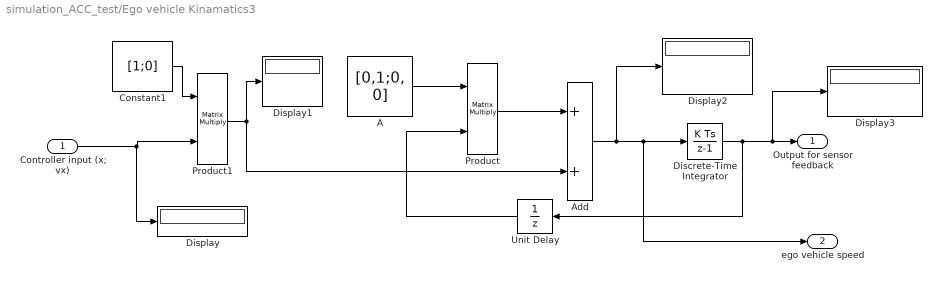
== system simulation_ACC_test/Ego vehicle Kinamatics3 ==
  Controller input (x; vx) : Inport
  A : Constant  Value=[0,1;0, 0]  VectorParams1D=off
  Add : Sum
  Constant1 : Constant  Value=[1;0]  VectorParams1D=off
  Discrete-Time Integrator : DiscreteIntegrator  InitialCondition=[0;0]  SampleTime=-1  ICPrevOutput=DiscIntNeverNeededParam  ICPrevScaledInput=DiscIntNeverNeededParam
  Display{,1..3} (4 alike) : Display
  Product : Product  Multiplication=Matrix(*)
  Product1 : Product  Multiplication=Matrix(*)
  Unit Delay : UnitDelay  SampleTime=-1
  Output for sensor feedback : Outport
  ego vehicle speed : Outport  Port=2
  wires:
  Discrete-Time Integrator/1 -> Unit Delay/1, Display3/1, Output for sensor feedback/1
  A/1 -> Product/1
  Controller input (x; vx)/1 -> Display/1, Product1/2
  Product1/1 -> Display1/1, Add/2
  Add/1 -> Display2/1, ego vehicle speed/1, Discrete-Time Integrator/1
  Product/1 -> Add/1
  Constant1/1 -> Product1/1
  Unit Delay/1 -> Product/2

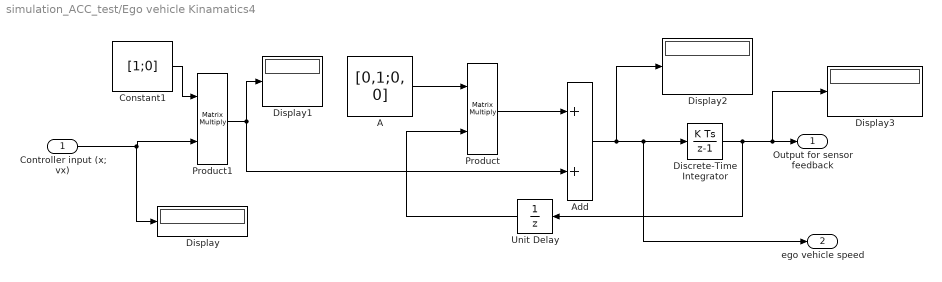
== system simulation_ACC_test/Ego vehicle Kinamatics4 ==
  Controller input (x; vx) : Inport
  A : Constant  Value=[0,1;0, 0]  VectorParams1D=off
  Add : Sum
  Constant1 : Constant  Value=[1;0]  VectorParams1D=off
  Discrete-Time Integrator : DiscreteIntegrator  InitialCondition=[0;0]  SampleTime=-1  ICPrevOutput=DiscIntNeverNeededParam  ICPrevScaledInput=DiscIntNeverNeededParam
  Display{,1..3} (4 alike) : Display
  Product : Product  Multiplication=Matrix(*)
  Product1 : Product  Multiplication=Matrix(*)
  Unit Delay : UnitDelay  SampleTime=-1
  Output for sensor feedback : Outport
  ego vehicle speed : Outport  Port=2
  wires:
  Discrete-Time Integrator/1 -> Unit Delay/1, Display3/1, Output for sensor feedback/1
  A/1 -> Product/1
  Controller input (x; vx)/1 -> Display/1, Product1/2
  Product1/1 -> Display1/1, Add/2
  Add/1 -> Display2/1, ego vehicle speed/1, Discrete-Time Integrator/1
  Product/1 -> Add/1
  Constant1/1 -> Product1/1
  Unit Delay/1 -> Product/2

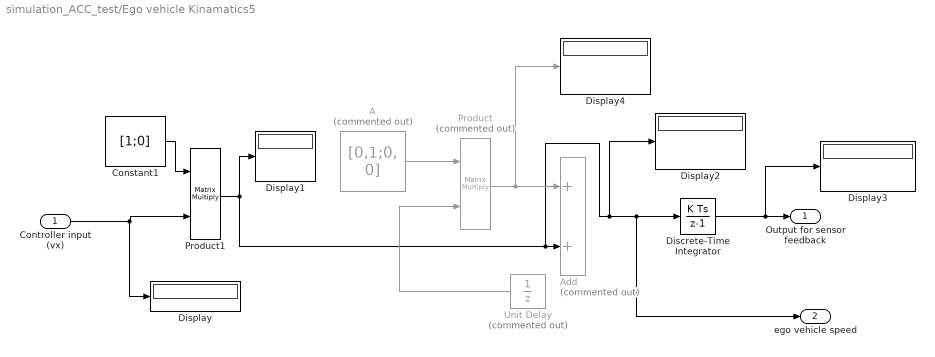
== system simulation_ACC_test/Ego vehicle Kinamatics5 ==
  Controller input (vx) : Inport
  A : Constant  Commented=on  Value=[0,1;0, 0]  VectorParams1D=off
  Add : Sum  Commented=on
  Constant1 : Constant  Value=[1;0]  VectorParams1D=off
  Discrete-Time Integrator : DiscreteIntegrator  InitialCondition=[0;0]  SampleTime=-1  ICPrevOutput=DiscIntNeverNeededParam  ICPrevScaledInput=DiscIntNeverNeededParam
  Display{,1..4} (5 alike) : Display
  Product : Product  Commented=on  Multiplication=Matrix(*)
  Product1 : Product  Multiplication=Matrix(*)
  Unit Delay : UnitDelay  Commented=on  SampleTime=-1
  Output for sensor feedback : Outport
  ego vehicle speed : Outport  Port=2
  wires:
  Discrete-Time Integrator/1 -> Display3/1, Output for sensor feedback/1
  A/1 -> Product/1
  Controller input (vx)/1 -> Display/1, Product1/2
  Product1/1 -> Display1/1, Display2/1, ego vehicle speed/1, Discrete-Time Integrator/1, Add/2
  Product/1 -> Display4/1, Add/1
  Constant1/1 -> Product1/1
  Unit Delay/1 -> Product/2

== system simulation_ACC_test/LDS sensor1 ==
  Traject. input : Inport
  AWGN Channel : commchan3/AWGN Channel  InputProcessing=Columns as channels (frame based)  seed=67  noiseMode="Signal to noise ratio  (SNR)"  EbNodB=100  EsNodB=10  SNRdB=27  bitsPerSym=1  Ps=1  Tsym=0.4  variance=1
  C : Constant  Value="[1, 0;    0, 1]"  VectorParams1D=off
  Product2 : Product  Multiplication=Matrix(*)
  Scope4 : Scope
  Scope7 : Scope
  Act lead vehicle speed : Outport
  Sensor Output : Outport  Port=2
  wires:
  Product2/1 -> Act lead vehicle speed/1, AWGN Channel/1, Scope7/1  "Actual Lead vehicle speed"
  C/1 -> Product2/1
  Traject. input/1 -> Product2/2, Scope4/1  "Trajectory input"
  AWGN Channel/1 -> Sensor Output/1  "Sensor output"

== system simulation_ACC_test/LDS sensor2 ==
  Traject. input : Inport
  AWGN Channel : commchan3/AWGN Channel  InputProcessing=Columns as channels (frame based)  seed=67  noiseMode="Signal to noise ratio  (SNR)"  EbNodB=100  EsNodB=10  SNRdB=27  bitsPerSym=1  Ps=1  Tsym=0.4  variance=1
  C : Constant  Commented=on  Value=[1, 0]  VectorParams1D=off
  Scope4 : Scope
  Scope7 : Scope
  sensor rel. distance : Outport
  Sensor Output : Outport  Port=2
  wires:
  Traject. input/1 -> sensor rel. distance/1, AWGN Channel/1, Scope7/1, Scope4/1  "Trajectory input"
  AWGN Channel/1 -> Sensor Output/1  "Sensor output"

== system simulation_ACC_test/LDS sensor3 ==
  Traject. input : Inport
  AWGN Channel : commchan3/AWGN Channel  InputProcessing=Columns as channels (frame based)  seed=67  noiseMode="Signal to noise ratio  (SNR)"  EbNodB=100  EsNodB=10  SNRdB=27  bitsPerSym=1  Ps=1  Tsym=0.4  variance=1
  C : Constant  Value="[1, 0;    0, 1]"  VectorParams1D=off
  Product2 : Product  Multiplication=Matrix(*)
  Scope4 : Scope
  Scope7 : Scope
  Act lead vehicle speed : Outport
  Sensor Output : Outport  Port=2
  wires:
  Product2/1 -> Act lead vehicle speed/1, AWGN Channel/1, Scope7/1  "Actual Lead vehicle speed"
  C/1 -> Product2/1
  Traject. input/1 -> Product2/2, Scope4/1  "Trajectory input"
  AWGN Channel/1 -> Sensor Output/1  "Sensor output"

== system simulation_ACC_test/LDS sensor4 ==
  Traject. input : Inport
  AWGN Channel : commchan3/AWGN Channel  InputProcessing=Columns as channels (frame based)  seed=67  noiseMode="Signal to noise ratio  (SNR)"  EbNodB=100  EsNodB=10  SNRdB=27  bitsPerSym=1  Ps=1  Tsym=0.4  variance=1
  C : Constant  Value="[1, 0;    0, 1]"  VectorParams1D=off
  Product2 : Product  Multiplication=Matrix(*)
  Scope4 : Scope
  Scope7 : Scope
  Act lead vehicle speed : Outport
  Sensor Output : Outport  Port=2
  wires:
  Product2/1 -> Act lead vehicle speed/1, AWGN Channel/1, Scope7/1  "Actual Lead vehicle speed"
  C/1 -> Product2/1
  Traject. input/1 -> Product2/2, Scope4/1  "Trajectory input"
  AWGN Channel/1 -> Sensor Output/1  "Sensor output"

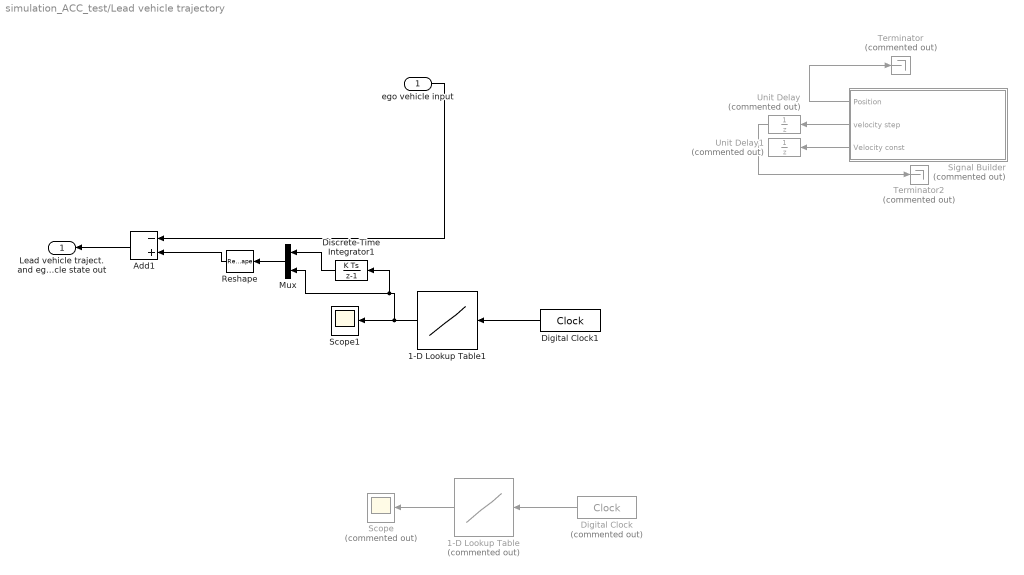
== system simulation_ACC_test/Lead vehicle trajectory ==
  ego vehicle input : Inport
  1-D Lookup Table : Lookup_n-D  Commented=on  NumberOfTableDimensions=1  BreakpointsForDimension1=timebpt  Table=lead_bot_vel_vari  ExtrapMethod=Clip  InternalRulePriority=Speed  RndMeth=Simplest  InputSameDT=on
  1-D Lookup Table1 : Lookup_n-D  NumberOfTableDimensions=1  BreakpointsForDimension1=timebpt  Table=lead_bot_vel_vari_const  ExtrapMethod=Clip  InternalRulePriority=Speed  RndMeth=Simplest  InputSameDT=on
  Add1 : Sum  Inputs=-+
  Digital Clock : DigitalClock  Commented=on  SampleTime=0.4
  Digital Clock1 : DigitalClock  SampleTime=0.4
  Discrete-Time Integrator1 : DiscreteIntegrator  SampleTime=-1  ICPrevOutput=DiscIntNeverNeededParam  ICPrevScaledInput=DiscIntNeverNeededParam
  Mux : Mux  Inputs=2
  Reshape : Reshape  OutputDimensionality=Column vector (2-D)
  Scope : Scope  Commented=on
  Scope1 : Scope
  Signal Builder : Subsystem  Tag=STV Subsys  Commented=on  LoadFcn=sigbuilder_block('load');  StartFcn=sigbuilder_block('start');  StopFcn=sigbuilder_block('stop');  ClipboardFcn=sigbuilder_block('clipboard');  mask(Sigbuilder block){tuvar=[0:10]}
      mask help: Simulink:masks:SigbuilderBlock_MD
      mask init:
      | if ~strcmp(get_param(bdroot(gcbh),'SimulationStatus'),'stopped') tuvar = sigbuilder_block('maskInit'); end
      settings: CopyFcn=sigbuilder_block('copy');  DeleteFcn=sigbuilder_block('delete');  ModelCloseFcn=sigbuilder_block('modelClose');  PreSaveFcn=sigbuilder_block('preSave');  PauseFcn=sigbuilder_block('pause');  ContinueFcn=sigbuilder_block('continue');  NameChangeFcn=sigbuilder_block('namechange');  OpenFcn=sigbuilder_block('open',[439.5 191.25 550.5 399.75 ]);  CloseFcn=sigbuilder_block('close');
      mask Display: plot(0, 0, 100, 100,[2, 2, 32, 32, 2], [68, 8, 8, 68, 68],[32, 2], [38, 38], [32, 19, 2],[53, 60, 44], [32, 17, 17, 2],[16, 16, 31, 31]);txt = getActiveGroup(gcbh);text(2, 100, txt,'verticalAlignment', 'top');
  Terminator : Terminator  Commented=on
  Terminator2 : Terminator  Commented=on
  Unit Delay : UnitDelay  Commented=on  SampleTime=-1
  Unit Delay1 : UnitDelay  Commented=on  SampleTime=-1
  Lead vehicle traject. and ego vehicle state out : Outport
  wires:
  Signal Builder/1(Position) -> Terminator/1
  Mux/1 -> Reshape/1
  Reshape/1 -> Add1/2
  Discrete-Time Integrator1/1 -> Mux/1
  ego vehicle input/1 -> Add1/1
  Add1/1 -> Lead vehicle traject. and ego vehicle state out/1
  Signal Builder/3(Velocity const) -> Unit Delay1/1
  Signal Builder/2(velocity step) -> Unit Delay/1
  Unit Delay/1 -> Terminator2/1
  Digital Clock/1 -> 1-D Lookup Table/1
  1-D Lookup Table/1 -> Scope/1
  Digital Clock1/1 -> 1-D Lookup Table1/1
  1-D Lookup Table1/1 -> Discrete-Time Integrator1/1, Mux/2, Scope1/1

== system simulation_ACC_test/Lead vehicle trajectory1 ==
  ego vehicle input : Inport
  Add1 : Sum  Inputs=-+
  Discrete-Time Integrator1 : DiscreteIntegrator  InitialCondition=0.6  SampleTime=-1  ICPrevOutput=DiscIntNeverNeededParam  ICPrevScaledInput=DiscIntNeverNeededParam
  Display : Display
  Display1 : Display
  Mux : Mux  Inputs=2
  Reshape : Reshape  OutputDimensionality=Column vector (2-D)
  Signal Builder : Subsystem  Tag=STV Subsys  LoadFcn=sigbuilder_block('load');  StartFcn=sigbuilder_block('start');  StopFcn=sigbuilder_block('stop');  ClipboardFcn=sigbuilder_block('clipboard');  mask(Sigbuilder block){tuvar=[0:10]}
      mask help: Simulink:masks:SigbuilderBlock_MD
      mask init:
      | if ~strcmp(get_param(bdroot(gcbh),'SimulationStatus'),'stopped') tuvar = sigbuilder_block('maskInit'); end
      settings: CopyFcn=sigbuilder_block('copy');  DeleteFcn=sigbuilder_block('delete');  ModelCloseFcn=sigbuilder_block('modelClose');  PreSaveFcn=sigbuilder_block('preSave');  PauseFcn=sigbuilder_block('pause');  ContinueFcn=sigbuilder_block('continue');  NameChangeFcn=sigbuilder_block('namechange');  OpenFcn=sigbuilder_block('open',[439.5 191.25 550.5 399.75 ]);  CloseFcn=sigbuilder_block('close');
      mask Display: plot(0, 0, 100, 100,[2, 2, 32, 32, 2], [68, 8, 8, 68, 68],[32, 2], [38, 38], [32, 19, 2],[53, 60, 44], [32, 17, 17, 2],[16, 16, 31, 31]);txt = getActiveGroup(gcbh);text(2, 100, txt,'verticalAlignment', 'top');
  Terminator : Terminator
  Terminator2 : Terminator
  Lead vehicle traject. and ego vehicle state out : Outport
  wires:
  Signal Builder/3(Velocity const) -> Discrete-Time Integrator1/1, Mux/2
  Signal Builder/1(Position) -> Terminator/1
  Mux/1 -> Reshape/1
  Signal Builder/2(velocity step) -> Terminator2/1
  Reshape/1 -> Display1/1, Add1/2
  Discrete-Time Integrator1/1 -> Mux/1
  ego vehicle input/1 -> Add1/1, Display/1
  Add1/1 -> Lead vehicle traject. and ego vehicle state out/1

== system simulation_ACC_test/Lead vehicle trajectory2 ==
  ego vehicle input : Inport
  Add1 : Sum  Inputs=-+
  Discrete-Time Integrator1 : DiscreteIntegrator  InitialCondition=0.6  SampleTime=-1  ICPrevOutput=DiscIntNeverNeededParam  ICPrevScaledInput=DiscIntNeverNeededParam
  Display : Display
  Display1 : Display
  Mux : Mux  Inputs=2
  Reshape : Reshape  OutputDimensionality=Column vector (2-D)
  Signal Builder : Subsystem  Tag=STV Subsys  LoadFcn=sigbuilder_block('load');  StartFcn=sigbuilder_block('start');  StopFcn=sigbuilder_block('stop');  ClipboardFcn=sigbuilder_block('clipboard');  mask(Sigbuilder block){tuvar=[0:10]}
      mask help: Simulink:masks:SigbuilderBlock_MD
      mask init:
      | if ~strcmp(get_param(bdroot(gcbh),'SimulationStatus'),'stopped') tuvar = sigbuilder_block('maskInit'); end
      settings: CopyFcn=sigbuilder_block('copy');  DeleteFcn=sigbuilder_block('delete');  ModelCloseFcn=sigbuilder_block('modelClose');  PreSaveFcn=sigbuilder_block('preSave');  PauseFcn=sigbuilder_block('pause');  ContinueFcn=sigbuilder_block('continue');  NameChangeFcn=sigbuilder_block('namechange');  OpenFcn=sigbuilder_block('open',[439.5 191.25 550.5 399.75 ]);  CloseFcn=sigbuilder_block('close');
      mask Display: plot(0, 0, 100, 100,[2, 2, 32, 32, 2], [68, 8, 8, 68, 68],[32, 2], [38, 38], [32, 19, 2],[53, 60, 44], [32, 17, 17, 2],[16, 16, 31, 31]);txt = getActiveGroup(gcbh);text(2, 100, txt,'verticalAlignment', 'top');
  Terminator : Terminator
  Terminator2 : Terminator
  Lead vehicle traject. and ego vehicle state out : Outport
  wires:
  Signal Builder/3(Velocity const) -> Discrete-Time Integrator1/1, Mux/2
  Signal Builder/1(Position) -> Terminator/1
  Mux/1 -> Reshape/1
  Signal Builder/2(velocity step) -> Terminator2/1
  Reshape/1 -> Display1/1, Add1/2
  Discrete-Time Integrator1/1 -> Mux/1
  ego vehicle input/1 -> Add1/1, Display/1
  Add1/1 -> Lead vehicle traject. and ego vehicle state out/1

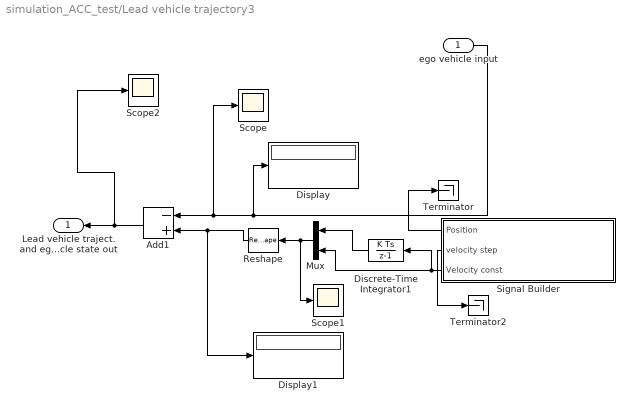
== system simulation_ACC_test/Lead vehicle trajectory3 ==
  ego vehicle input : Inport
  Add1 : Sum  Inputs=-+
  Discrete-Time Integrator1 : DiscreteIntegrator  InitialCondition=0.6  SampleTime=-1  ICPrevOutput=DiscIntNeverNeededParam  ICPrevScaledInput=DiscIntNeverNeededParam
  Display : Display
  Display1 : Display
  Mux : Mux  Inputs=2
  Reshape : Reshape  OutputDimensionality=Column vector (2-D)
  Scope : Scope
  Scope1 : Scope
  Scope2 : Scope
  Signal Builder : Subsystem  Tag=STV Subsys  LoadFcn=sigbuilder_block('load');  StartFcn=sigbuilder_block('start');  StopFcn=sigbuilder_block('stop');  ClipboardFcn=sigbuilder_block('clipboard');  mask(Sigbuilder block){tuvar=[0:10]}
      mask help: Simulink:masks:SigbuilderBlock_MD
      mask init:
      | if ~strcmp(get_param(bdroot(gcbh),'SimulationStatus'),'stopped') tuvar = sigbuilder_block('maskInit'); end
      settings: CopyFcn=sigbuilder_block('copy');  DeleteFcn=sigbuilder_block('delete');  ModelCloseFcn=sigbuilder_block('modelClose');  PreSaveFcn=sigbuilder_block('preSave');  PauseFcn=sigbuilder_block('pause');  ContinueFcn=sigbuilder_block('continue');  NameChangeFcn=sigbuilder_block('namechange');  OpenFcn=sigbuilder_block('open',[366 236.25 550.5 399.75 ]);  CloseFcn=sigbuilder_block('close');
      mask Display: plot(0, 0, 100, 100,[2, 2, 32, 32, 2], [68, 8, 8, 68, 68],[32, 2], [38, 38], [32, 19, 2],[53, 60, 44], [32, 17, 17, 2],[16, 16, 31, 31]);txt = getActiveGroup(gcbh);text(2, 100, txt,'verticalAlignment', 'top');
  Terminator : Terminator
  Terminator2 : Terminator
  Lead vehicle traject. and ego vehicle state out : Outport
  wires:
  Signal Builder/1(Position) -> Terminator/1
  Mux/1 -> Scope1/1, Reshape/1
  Reshape/1 -> Display1/1, Add1/2
  Discrete-Time Integrator1/1 -> Mux/1
  ego vehicle input/1 -> Scope/1, Add1/1, Display/1
  Add1/1 -> Scope2/1, Lead vehicle traject. and ego vehicle state out/1
  Signal Builder/3(Velocity const) -> Mux/2, Discrete-Time Integrator1/1
  Signal Builder/2(velocity step) -> Terminator2/1
